simulink model "Load_Current_Limits"  (R2024b)
settings: configuration reference "ConfigSet_Sim_ASW" (kept outside this file)
model workspace (MAT data in the model file):
  TsModel = 0.1
undefined symbols (not defined in the file): Curr_Test_Load, Voltage_Test_Vector
libraries: simulink x1
settings Model: DataDictionary=LocalDataD_Load_Current_Limits.sldd  ExtModeTrigDuration=8  Creator=vivekr  LastModifiedBy=vlenzi
settings ConfigSetRef: SourceName=ConfigSet_Sim_ASW

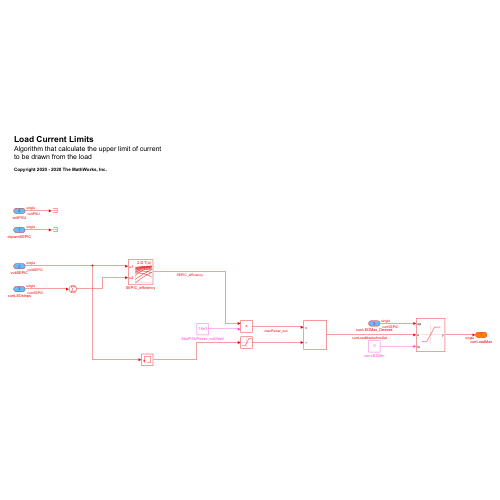
[thumbnail: Simulink's stored preview of the top-level diagram]
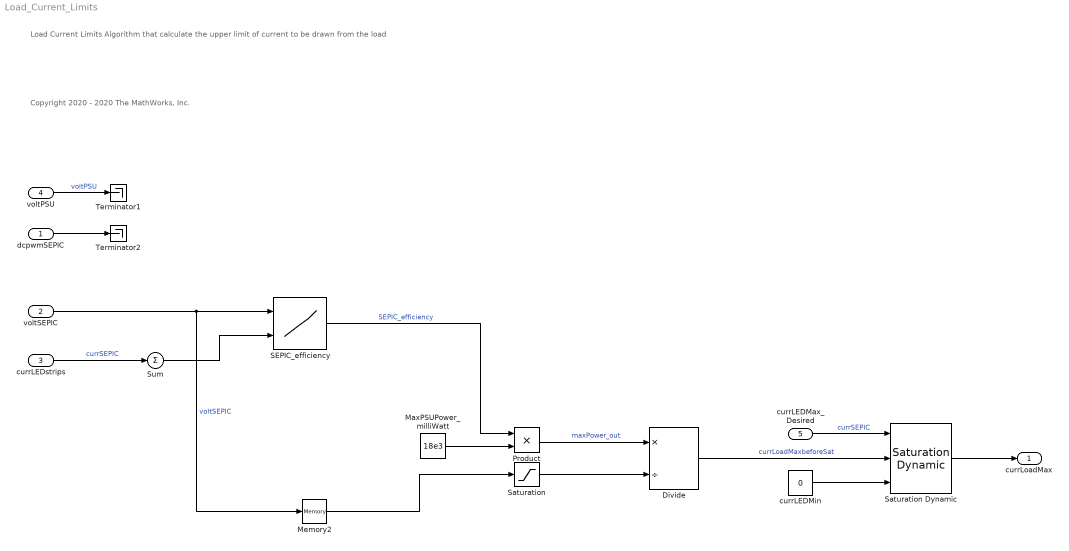
== system Load_Current_Limits ==
  note: Load Current Limits
      | Algorithm that calculate the upper limit of current to be drawn from the load
  note: Copyright 2020 - 2020 The MathWorks, Inc.
  dcpwmSEPIC : Inport  OutDataTypeStr=single  Unit=1  PortDimensions=1  SampleTime=TsModel
  voltSEPIC : Inport  Port=2  OutDataTypeStr=single  Unit=V  PortDimensions=1  SampleTime=TsModel
  currLEDstrips : Inport  Port=3  OutDataTypeStr=single  Unit=mA  PortDimensions=6  SampleTime=TsModel
  voltPSU : Inport  Port=4  OutDataTypeStr=single  Unit=V  PortDimensions=1  SampleTime=TsModel
  currLEDMax_Desired : Inport  Port=5  OutDataTypeStr=single  Unit=mA  PortDimensions=1  SampleTime=TsModel
  Divide : Product  Inputs=*/
  MaxPSUPower_milliWatt : Constant  Value=18e3  OutDataTypeStr=single  SampleTime=-1
  Memory2 : Memory
  Product : Product
  SEPIC_efficiency : Lookup_n-D  BreakpointsForDimension1=Voltage_Test_Vector  BreakpointsForDimension2=Curr_Test_Load  Table=effMatrix'  ExtrapMethod=Clip  UseLastTableValue=on  InternalRulePriority=Speed  RndMeth=Simplest
      settings: InputPortMap=u0,u1
  Saturation : Saturate  UpperLimit=50  LowerLimit=1e-3
  Saturation Dynamic : simulink/Discontinuities/Saturation Dynamic  OutMin=[]  OutMax=[]  OutDataTypeStr=Inherit: Same as second input  OutDataType=fixdt(1, 16)  OutScaling=2^-10  DoSatur=off
  Sum : Sum  Inputs=+
  Terminator1 : Terminator
  Terminator2 : Terminator
  currLEDMin : Constant  Value=0  OutDataTypeStr=single  SampleTime=-1
  currLoadMax : Outport  OutDataTypeStr=single  Unit=mA  PortDimensions=1  SampleTime=TsModel
  wires:
  voltPSU/1 -> Terminator1/1  "voltPSU"
  voltSEPIC/1 -> Memory2/1, SEPIC_efficiency/1  "voltSEPIC"
  MaxPSUPower_milliWatt/1 -> Product/2
  Saturation/1 -> Divide/2
  dcpwmSEPIC/1 -> Terminator2/1
  currLEDstrips/1 -> Sum/1  "currSEPIC"
  Memory2/1 -> Saturation/1
  Divide/1 -> Saturation Dynamic/2  "currLoadMaxbeforeSat"
  SEPIC_efficiency/1 -> Product/1  "SEPIC_efficiency"
  Saturation Dynamic/1 -> currLoadMax/1
  currLEDMax_Desired/1 -> Saturation Dynamic/1  "currSEPIC"
  currLEDMin/1 -> Saturation Dynamic/3
  Sum/1 -> SEPIC_efficiency/2
  Product/1 -> Divide/1  "maxPower_out"
